simulink model "untitled"  (R2020b)
settings: Solver=FixedStepDiscrete  StartTime=0.0  StopTime=500000.0  FixedStep=1  RelTol=1e-3
settings Model: Creator=Nic  LastModifiedBy=Nic

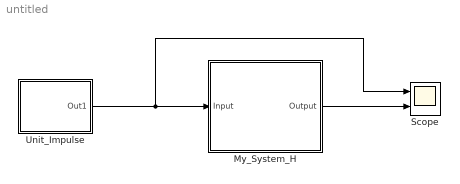
== system untitled ==
  My_System_H : Subsystem
  Scope : Scope  NumInputPorts=2
  Unit_Impulse : Subsystem
  wires:
  My_System_H/1(Output) -> Scope/2
  Unit_Impulse/1(Out1) -> My_System_H/1(Input), Scope/1

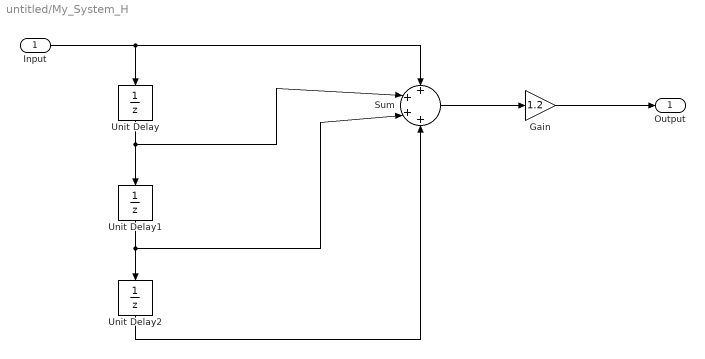
== system untitled/My_System_H ==
  Input : Inport
  Gain : Gain  Gain=1.2
  Sum : Sum  Inputs=++++
  Unit Delay : UnitDelay  SampleTime=-1  HasFrameUpgradeWarning=on
  Unit Delay1 : UnitDelay  SampleTime=-1  HasFrameUpgradeWarning=on
  Unit Delay2 : UnitDelay  SampleTime=-1  HasFrameUpgradeWarning=on
  Output : Outport
  wires:
  Unit Delay1/1 -> Sum/3, Unit Delay2/1
  Sum/1 -> Gain/1
  Input/1 -> Sum/1, Unit Delay/1
  Unit Delay/1 -> Unit Delay1/1, Sum/2
  Unit Delay2/1 -> Sum/4
  Gain/1 -> Output/1

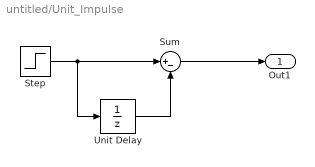
== system untitled/Unit_Impulse ==
  Step : Step  SampleTime=0
  Sum : Sum  Inputs=|+-
  Unit Delay : UnitDelay  SampleTime=-1  HasFrameUpgradeWarning=on
  Out1 : Outport
  wires:
  Step/1 -> Unit Delay/1, Sum/1
  Unit Delay/1 -> Sum/2
  Sum/1 -> Out1/1
